simulink model "Strecke_v1"  (R2026a)
settings: Solver=VariableStepAuto
values from neighbouring files (symbols this model uses):
  b = 0.1    [StreckeEntwurf_nichtlineare.m]    (also in StreckeEntwurf_ss.m)
  g = 9.81    [StreckeEntwurf_nichtlineare.m]    (also in StreckeEntwurf_ss.m; scratchpad.m = 9.8)
  l = 1    [StreckeEntwurf_nichtlineare.m]    (also in StreckeEntwurf_ss.m = 0.3)
  M = 1    [StreckeEntwurf_nichtlineare.m]    (also in StreckeEntwurf_ss.m = 0.5)
  m = 1    [StreckeEntwurf_nichtlineare.m]    (also in StreckeEntwurf_ss.m = 0.2)
settings Model: Creator=me  LastModifiedBy=me

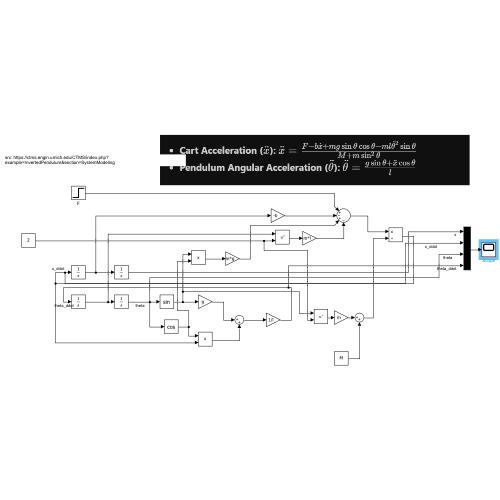
[thumbnail: Simulink's stored preview of the top-level diagram]
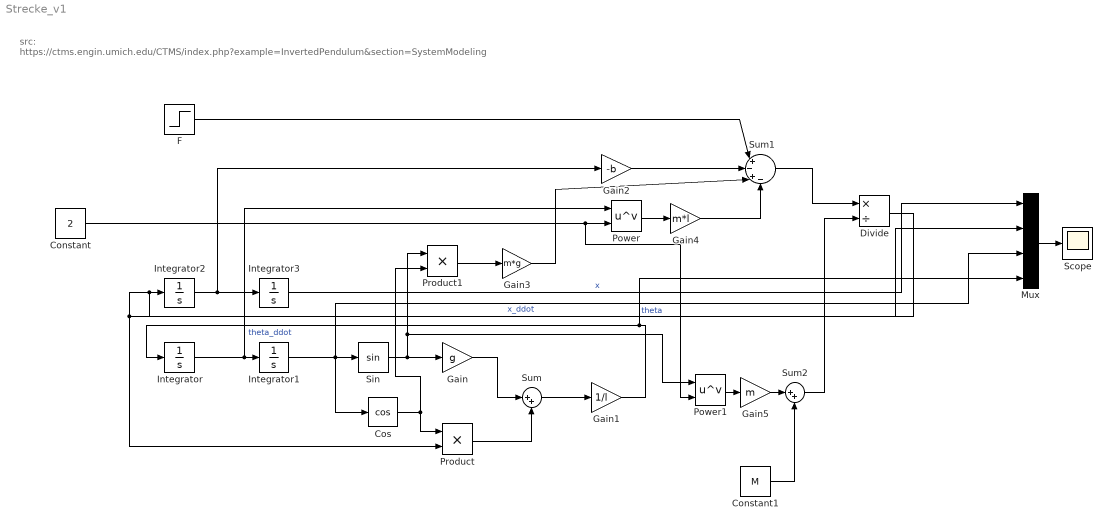
== system Strecke_v1 ==
  note: src: https://ctms.engin.umich.edu/CTMS/index.php?example=InvertedPendulum&section=SystemModeling
  Constant : Constant  Value=2
  Constant1 : Constant  Value=M
  Cos : Trigonometry  Operator=cos
  Divide : Product  Inputs=*/
  F : Step  SampleTime=0
  Gain : Gain  Gain=g
  Gain1 : Gain  Gain=1/l
  Gain2 : Gain  Gain=-b
  Gain3 : Gain  Gain=m*g
  Gain4 : Gain  Gain=m*l
  Gain5 : Gain  Gain=m
  Integrator{,1..3} (4 alike) : Integrator
  Mux : Mux
  Power : Math  Operator=pow
  Power1 : Math  Operator=pow
  Product : Product
  Product1 : Product
  Scope : Scope
      settings: ActiveDisplayYMinimum=-50907.58366610005  ActiveDisplayYMaximum=21005.3808531315
  Sin : Trigonometry
  Sum : Sum  Inputs=|++
  Sum1 : Sum  Inputs=|+-+-
  Sum2 : Sum  Inputs=|++
  wires:
  Integrator/1 -> Power/1, Integrator1/1
  Integrator1/1 -> Cos/1, Sin/1, Mux/3  "theta"
  Gain1/1 -> Mux/4, Integrator/1  "theta_ddot"
  Integrator2/1 -> Gain2/1, Integrator3/1
  Divide/1 -> Mux/2, Integrator2/1, Product/2  "x_ddot"
  Sin/1 -> Power1/1, Product1/1, Gain/1
  Cos/1 -> Product1/2, Product/1
  Gain/1 -> Sum/1
  Product/1 -> Sum/2
  Sum/1 -> Gain1/1
  F/1 -> Sum1/1
  Gain2/1 -> Sum1/2
  Product1/1 -> Gain3/1
  Gain3/1 -> Sum1/3
  Constant/1 -> Power/2, Power1/2
  Power/1 -> Gain4/1
  Gain4/1 -> Sum1/4
  Sum1/1 -> Divide/1
  Constant1/1 -> Sum2/2
  Gain5/1 -> Sum2/1
  Power1/1 -> Gain5/1
  Sum2/1 -> Divide/2
  Mux/1 -> Scope/1
  Integrator3/1 -> Mux/1  "x"
